simulink model "bounce"  (R2024b)
settings: Solver=ode15s  StartTime=0.0  StopTime=t_f  RelTol=1e-8
undefined symbols (not defined in the file): grav, mass, X_LF, X_LR, X_RF, X_RR
settings Model: Creator=yevge  LastModifiedBy=Yevgeniy Gorbachev

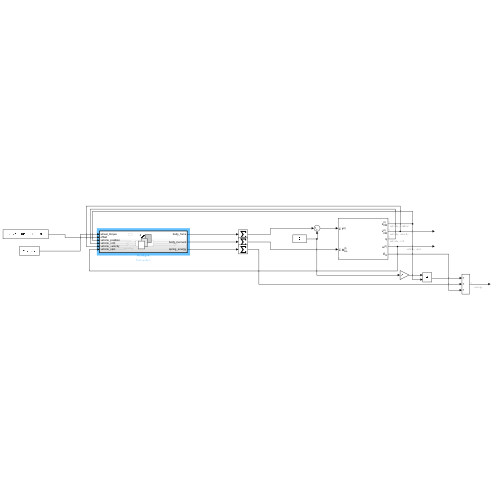
[thumbnail: Simulink's stored preview of the top-level diagram]
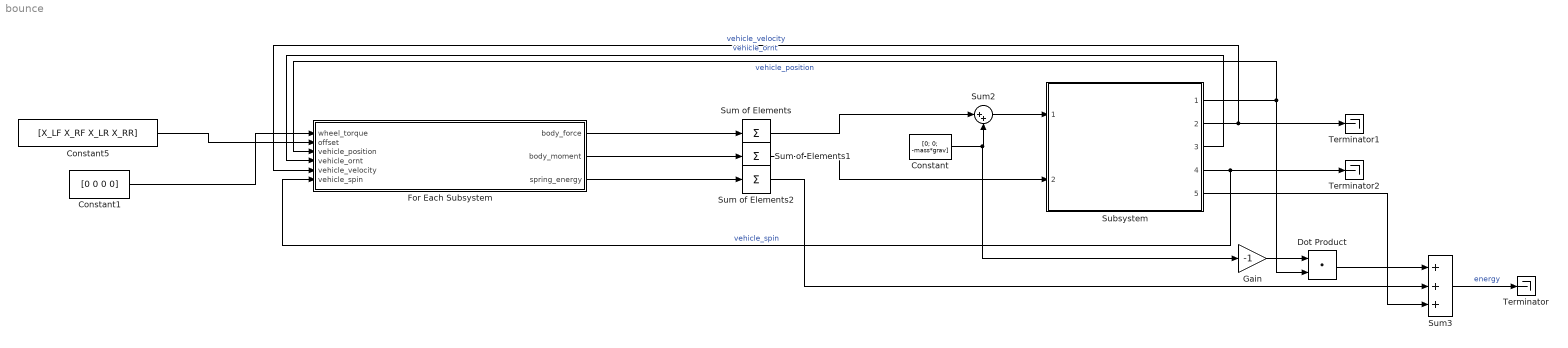
== system bounce ==
  Constant : Constant  Value=[0; 0; -mass*grav]
  Constant1 : Constant  Value=[0 0 0 0]
  Constant5 : Constant  Value=[X_LF X_RF X_LR X_RR]
  Dot Product : DotProduct  OutDataTypeStr=Inherit: Inherit via internal rule
  For Each Subsystem : Subsystem  TreatAsAtomicUnit=on
  Gain : Gain  Gain=-1
  Subsystem : Subsystem  ReferencedSubsystem=rigid_body_sixdof  pos_0=vehicle_pos_0  vel_0=vehicle_vel_0  ornt_0=vehicle_ornt_0  mass=mass  inertia=inertia  spin_0=vehicle_spin_0
  Sum of Elements : Sum  Inputs=+  CollapseMode=Specified dimension  CollapseDim=2
  Sum of Elements1 : Sum  Inputs=+  CollapseMode=Specified dimension  CollapseDim=2
  Sum of Elements2 : Sum  Inputs=+  CollapseMode=Specified dimension  CollapseDim=2
  Sum2 : Sum  Inputs=|++
  Sum3 : Sum  Inputs=3
  Terminator : Terminator
  Terminator1 : Terminator
  Terminator2 : Terminator
  wires:
  Constant/1 -> Gain/1, Sum2/2
  Subsystem/1 -> Dot Product/2, For Each Subsystem/3(vehicle_position)  "vehicle_position"
  Subsystem/2 -> For Each Subsystem/5(vehicle_velocity), Terminator1/1  "vehicle_velocity"
  Subsystem/4 -> For Each Subsystem/6(vehicle_spin), Terminator2/1  "vehicle_spin"
  Gain/1 -> Dot Product/1
  Dot Product/1 -> Sum3/1
  Subsystem/5 -> Sum3/3
  Sum3/1 -> Terminator/1  "energy"
  Constant5/1 -> For Each Subsystem/2(offset)
  For Each Subsystem/1(body_force) -> Sum of Elements/1
  For Each Subsystem/2(body_moment) -> Sum of Elements1/1
  For Each Subsystem/3(spring_energy) -> Sum of Elements2/1
  Sum of Elements/1 -> Sum2/1
  Sum of Elements1/1 -> Subsystem/2
  Sum of Elements2/1 -> Sum3/2
  Subsystem/3 -> For Each Subsystem/4(vehicle_ornt)  "vehicle_ornt"
  Sum2/1 -> Subsystem/1
  Constant1/1 -> For Each Subsystem/1(wheel_torque)

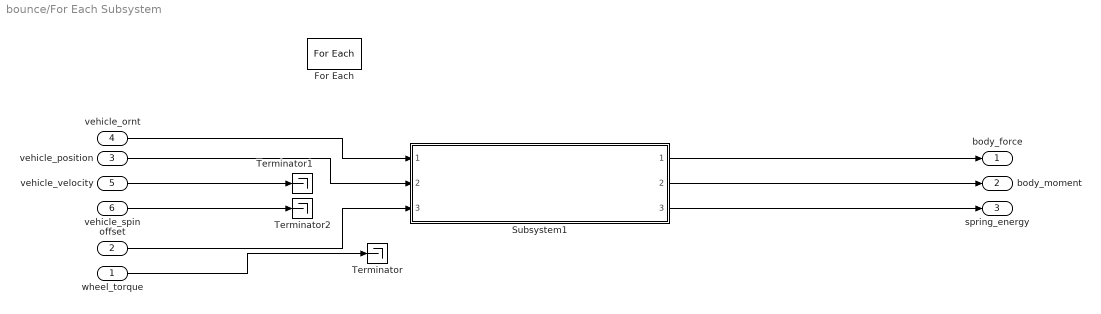
== system bounce/For Each Subsystem ==
  wheel_torque : Inport  Unit=N*m@torque  PortDimensions=[1 4]  Partition=on  PartitionDimension=2  PartitionWidth=1  PartitionOffset=0
  offset : Inport  Port=2  Unit=m  PortDimensions=[3 1]  Partition=on  PartitionDimension=2  PartitionWidth=1  PartitionOffset=0
  vehicle_position : Inport  Port=3  Unit=m  PortDimensions=[3 1]
  vehicle_ornt : Inport  Port=4  Unit=1  PortDimensions=[4 1]
  vehicle_velocity : Inport  Port=5
  vehicle_spin : Inport  Port=6
  For Each : ForEach  DisableCoverage=on
  Subsystem1 : Subsystem  ReferencedSubsystem=quarter_suspension
  Terminator : Terminator
  Terminator1 : Terminator
  Terminator2 : Terminator
  body_force : Outport  ConcatenationDimension=2
  body_moment : Outport  Port=2  ConcatenationDimension=2
  spring_energy : Outport  Port=3  ConcatenationDimension=2
  wires:
  offset/1 -> Subsystem1/3
  Subsystem1/1 -> body_force/1
  Subsystem1/2 -> body_moment/1
  Subsystem1/3 -> spring_energy/1
  vehicle_ornt/1 -> Subsystem1/1
  vehicle_position/1 -> Subsystem1/2
  wheel_torque/1 -> Terminator/1
  vehicle_velocity/1 -> Terminator1/1
  vehicle_spin/1 -> Terminator2/1
